simulink model "LaneFollowingController"  (R2023b)
settings: Solver=FixedStepDiscrete  StartTime=0.0  StopTime=inf  RelTol=1e-3  EnableMultiTasking=on
undefined symbols (not defined in the file): BrStatus, driver_decel, FB_decel, headwayOffset, max_ac, max_dc, PB1_decel, PB2_decel, PredictionHorizon, stopVelThreshold, time_gap, timeMargin, timeToReact, Ts
libraries: mpcadaslib x1
settings Model: Creator=The MathWorks, Inc.  LastModifiedBy=The MathWorks, Inc.
settings SolverCC: AlgebraicLoopSolver=TrustRegion  MaxZcPerStep=1
settings DataIOCC: SaveOutput=off  SaveTime=off  ReturnWorkspaceOutputs=off
settings OptimizationCC: DefaultParameterBehavior=Inlined  InlineInvariantSignals=on  EnhancedBackFolding=on  PassReuseOutputArgsAs=Individual arguments  ZeroExternalMemoryAtStartup=off  ZeroInternalMemoryAtStartup=off  EfficientFloat2IntCast=on  OptimizeBlockOrder=speed  DifferentSizesBufferReuse=on  OptimizationCustomize=off  EfficientTunableParamExpr=on
settings DebuggingCC: ParameterPrecisionLossMsg=none  ParameterTunabilityLossMsg=error  UnconnectedInputMsg=warning  UnconnectedOutputMsg=warning  UnconnectedLineMsg=warning  PregeneratedLibrarySubsystemCodeDiagnostic=none  SubsystemReferenceDiagnosticForUnitTest=warning  ArithmeticOperatorsInVariantConditions=warning
settings HardwareCC: ProdLongLongMode=on
settings ModelReferenceCC: EnableRefExpFcnMdlSchedulingChecks=on  PropagateVarSize=During execution
settings SFSimCC: SimUseLocalCustomCode=off  SimTargetLang=C++
settings RTWCC: Description=Embedded Coder  SystemTargetFile=ert.tlc  TemplateMakefile=ert_default_tmf  RTWVerbose=off  RTWUseLocalCustomCode=off  BuildConfiguration=Faster Runs  IncludeHyperlinkInReport=on  CodeExecutionProfiling=on  CodeProfilingSaveOptions=AllData  TargetLang=C++  DLArmComputeVersion=19.05
settings CodeAppCC: ForceParamTrailComments=on  IgnoreCustomStorageClasses=off  MaxIdLength=127  OperatorAnnotations=on  SimulinkDataObjDesc=on  SFDataObjDesc=on  CustomSymbolStrGlobalVar=$N$M  CustomSymbolStrType=$N$M_T  CustomSymbolStrFcn=APV_$N$M$F  CustomSymbolStrMacro=$N$M  InsertBlockDesc=on
settings ERTTargetCC: TargetLangStandard=C++03 (ISO)  GenerateSampleERTMain=on  CombineSignalStateStructs=on  CodeInterfacePackaging=C++ class  SupportVariableSizeSignals=on  CastingMode=Standards  InlinedParameterPlacement=NonHierarchical  RootIOFormat=Structure reference  ERTCustomFileTemplate=example_file_process.tlc
settings ConfigComp: CovScope=ReferencedModels  CovIncludeTopModel=off

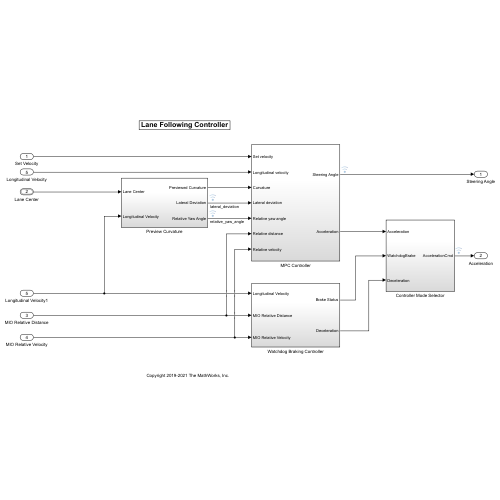
[thumbnail: Simulink's stored preview of the top-level diagram]
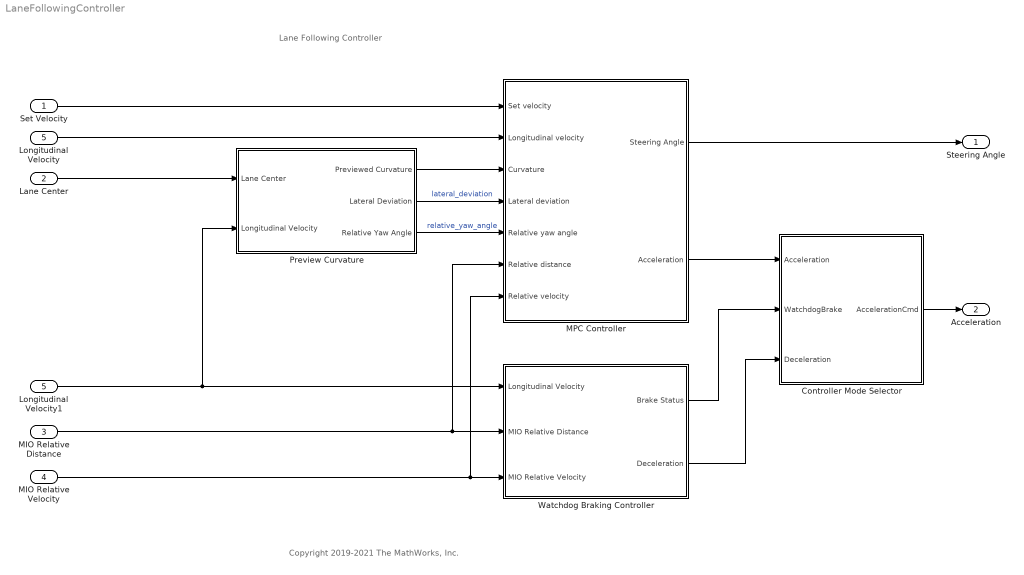
== system LaneFollowingController ==
  note: Copyright 2019-2021 The MathWorks, Inc.
  note: Lane Following Controller
  Set Velocity : Inport
  Lane Center : Inport  Port=2  OutDataTypeStr=Bus: BusLaneCenter
  MIO Relative Distance : Inport  Port=3
  MIO Relative Velocity : Inport  Port=4
  Longitudinal Velocity : Inport  Port=5
  Controller Mode Selector : Subsystem
  Longitudinal Velocity1 : InportShadow  Port=5
  MPC Controller : Subsystem
  Preview Curvature : Subsystem  VariantControl=v2
      settings: RTWFileNameOpts=Use function name
  Watchdog Braking Controller : Subsystem
  Steering Angle : Outport  PortDimensions=1  VectorParamsAs1DForOutWhenUnconnected=off
  Acceleration : Outport  Port=2  PortDimensions=1  VectorParamsAs1DForOutWhenUnconnected=off
  wires:
  Lane Center/1 -> Preview Curvature/1(Lane Center)
  Set Velocity/1 -> MPC Controller/1(Set velocity)
  Controller Mode Selector/1(AccelerationCmd) -> Acceleration/1
  Preview Curvature/3(Relative Yaw Angle) -> MPC Controller/5(Relative yaw angle)  "relative_yaw_angle"
  Longitudinal Velocity1/1 -> Preview Curvature/2(Longitudinal Velocity), Watchdog Braking Controller/1(Longitudinal Velocity)
  Watchdog Braking Controller/2(Deceleration) -> Controller Mode Selector/3(Deceleration)
  Watchdog Braking Controller/1(Brake Status) -> Controller Mode Selector/2(WatchdogBrake)
  Longitudinal Velocity/1 -> MPC Controller/2(Longitudinal velocity)
  MIO Relative Velocity/1 -> MPC Controller/7(Relative velocity), Watchdog Braking Controller/3(MIO Relative Velocity)
  Preview Curvature/2(Lateral Deviation) -> MPC Controller/4(Lateral deviation)  "lateral_deviation"
  MIO Relative Distance/1 -> Watchdog Braking Controller/2(MIO Relative Distance), MPC Controller/6(Relative distance)
  MPC Controller/1(Steering Angle) -> Steering Angle/1
  Preview Curvature/1(Previewed Curvature) -> MPC Controller/3(Curvature)
  MPC Controller/2(Acceleration) -> Controller Mode Selector/1(Acceleration)

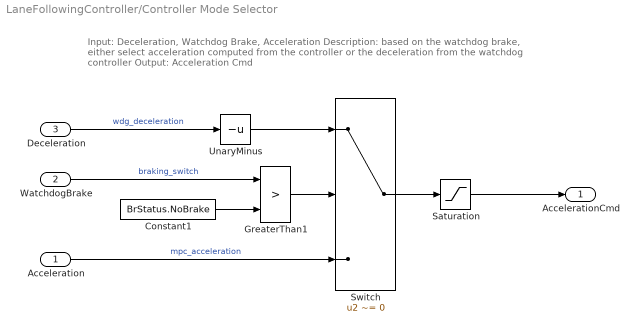
== system LaneFollowingController/Controller Mode Selector ==
  note: Input: Deceleration, Watchdog Brake, Acceleration
      | Description: based on the watchdog brake, either select acceleration computed from the controller or the deceleration from the watchdog controller
      | Output: Acceleration Cmd
  Acceleration : Inport
  WatchdogBrake : Inport  Port=2
  Deceleration : Inport  Port=3
  Constant1 : Constant  Value=BrStatus.NoBrake  OutDataTypeStr=Enum: BrStatus
  GreaterThan1 : RelationalOperator  Operator=>  RndMeth=Simplest  InputSameDT=off
  Saturation : Saturate  UpperLimit=max_ac  LowerLimit=max_dc
      settings: AttributesFormatString=|
      | %<UpperLimit>
      | %<LowerLimit>
  Switch : Switch  Criteria=u2 ~= 0  SaturateOnIntegerOverflow=off  InputSameDT=off
  UnaryMinus : UnaryMinus
  AccelerationCmd : Outport
  wires:
  Switch/1 -> Saturation/1
  WatchdogBrake/1 -> GreaterThan1/1  "braking_switch"
  UnaryMinus/1 -> Switch/1
  Deceleration/1 -> UnaryMinus/1  "wdg_deceleration"
  Saturation/1 -> AccelerationCmd/1
  Acceleration/1 -> Switch/3  "mpc_acceleration"
  Constant1/1 -> GreaterThan1/2
  GreaterThan1/1 -> Switch/2

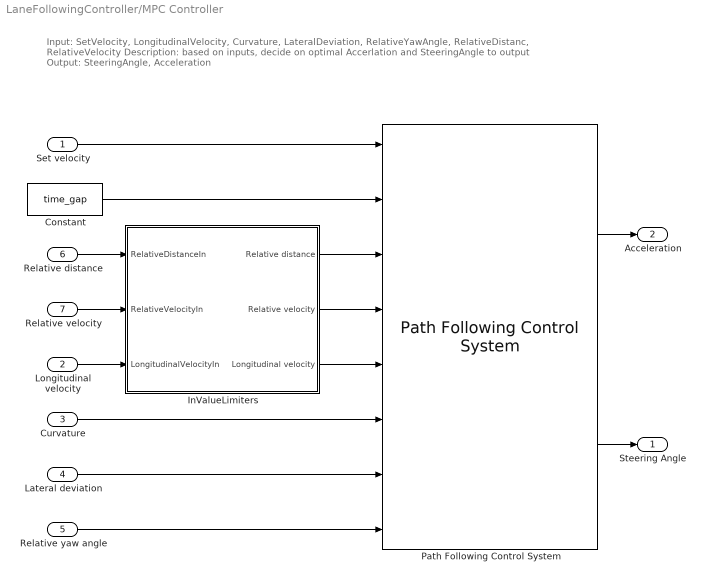
== system LaneFollowingController/MPC Controller ==
  note: Input: SetVelocity, LongitudinalVelocity, Curvature, LateralDeviation, RelativeYawAngle, RelativeDistanc, RelativeVelocity
      | Description: based on inputs, decide on optimal Accerlation and SteeringAngle to output
      | Output: SteeringAngle, Acceleration
  Set velocity : Inport
  Longitudinal velocity : Inport  Port=2
  Curvature : Inport  Port=3
  Lateral deviation : Inport  Port=4
  Relative yaw angle : Inport  Port=5
  Relative distance : Inport  Port=6
  Relative velocity : Inport  Port=7
  Constant : Constant  Value=time_gap
  InValueLimiters : Subsystem
  Path Following Control System : mpcadaslib/Path Following Control System  VariantControl=Variant2  ModelType=Use vehicle parameters  VehicleMass=m  VehicleYawInertia=Iz  LengthToFront=lf  LengthToRear=lr  FrontTireStiffness=Cf  RearTireStiffness=Cr  AccelTimeConstant=tau  EgoModelMatrixA=[-2,zeros(1,3);1,zeros(1,3);zeros(1,2),-4.4021,-12.4603;zeros(1,2),1.3913,-5.1868]  EgoModelMatrixB=[2,zeros(1,3);zeros(1,2),24.1270,15.8609]'  EgoModelMatrixC=[zeros(3,1),eye(3)]  InitialLongVel=v0_ego  TransportLag=Ts  spaceCtrl=on  DefaultSpacing=default_spacing  MinSteering=min_steer  umin_ext=off  MaxSteering=max_steer  umax_ext=off  MinAcceleration=min_ac  amin_ext=off  MaxAcceleration=max_ac  amax_ext=off  Ts=Ts  PredictionHorizon=PredictionHorizon  ControlHorizon=ControlHorizon  LongWeight=0.1  LateralWeight=1  AccelRateWeight=0.1  SteerRateWeight=0.1  suboptimal=off  maxiter=10  datatypeopt=double  optmode=off  trackmode=off
  Steering Angle : Outport  VectorParamsAs1DForOutWhenUnconnected=off
  Acceleration : Outport  Port=2  VectorParamsAs1DForOutWhenUnconnected=off
  wires:
  Constant/1 -> Path Following Control System/2
  Relative yaw angle/1 -> Path Following Control System/8
  Lateral deviation/1 -> Path Following Control System/7
  Curvature/1 -> Path Following Control System/6
  Set velocity/1 -> Path Following Control System/1
  Path Following Control System/2 -> Steering Angle/1
  Path Following Control System/1 -> Acceleration/1
  Longitudinal velocity/1 -> InValueLimiters/3(LongitudinalVelocityIn)
  Relative distance/1 -> InValueLimiters/1(RelativeDistanceIn)
  Relative velocity/1 -> InValueLimiters/2(RelativeVelocityIn)
  InValueLimiters/1(Relative distance) -> Path Following Control System/3
  InValueLimiters/2(Relative velocity) -> Path Following Control System/4
  InValueLimiters/3(Longitudinal velocity) -> Path Following Control System/5

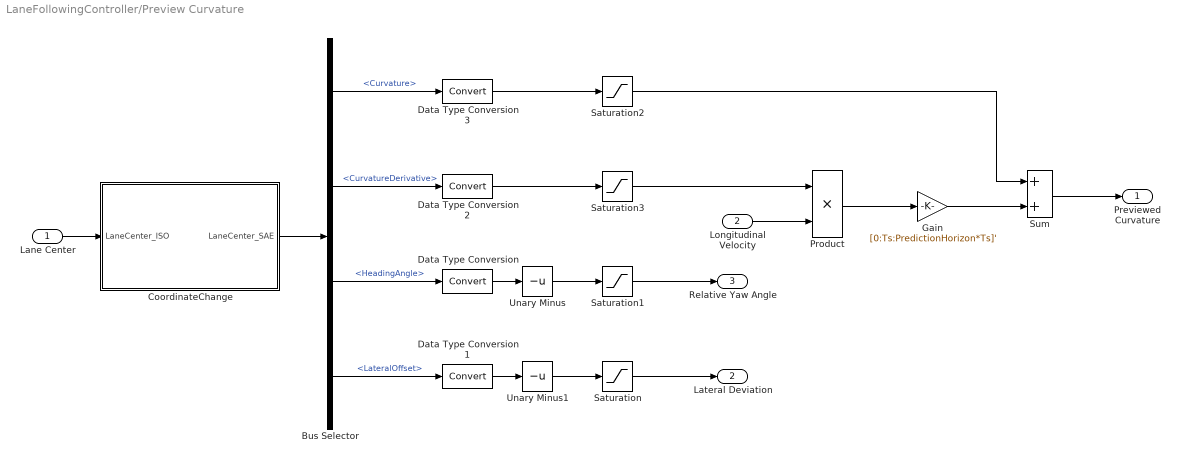
== system LaneFollowingController/Preview Curvature ==
  Lane Center : Inport
  Longitudinal Velocity : Inport  Port=2
  Bus Selector : BusSelector  OutputSignals=Curvature,CurvatureDerivative,HeadingAngle,LateralOffset
  CoordinateChange : Subsystem
  Data Type Conversion{,1..3} (4 alike) : DataTypeConversion  SaturateOnIntegerOverflow=off  RndMeth=Floor
  Gain : Gain  Gain=[0:Ts:PredictionHorizon*Ts]'
      settings: AttributesFormatString=|
      | ----------------------------------------
      | Gain = %<Gain>
  Product : Product
  Saturation : Saturate
      settings: AttributesFormatString=|
      | -------------------------------
      | UpperLimit = %<UpperLimit>
      | LowerLimit = %<LowerLimit>
  Saturation1 : Saturate  UpperLimit=0.6  LowerLimit=-0.6
      settings: AttributesFormatString=|
      | -------------------------------
      | UpperLimit = %<UpperLimit>
      | LowerLimit = %<LowerLimit>
  Saturation2 : Saturate  UpperLimit=0.15  LowerLimit=-0.15
      settings: AttributesFormatString=|
      | -------------------------------
      | UpperLimit = %<UpperLimit>
      | LowerLimit = %<LowerLimit>
  Saturation3 : Saturate  UpperLimit=0.06  LowerLimit=-0.06
      settings: AttributesFormatString=|
      | -------------------------------
      | UpperLimit = %<UpperLimit>
      | LowerLimit = %<LowerLimit>
  Sum : Sum
  Unary Minus : UnaryMinus
  Unary Minus1 : UnaryMinus
  Previewed Curvature : Outport  VectorParamsAs1DForOutWhenUnconnected=off
  Lateral Deviation : Outport  Port=2  VectorParamsAs1DForOutWhenUnconnected=off
  Relative Yaw Angle : Outport  Port=3  VectorParamsAs1DForOutWhenUnconnected=off
  wires:
  Lane Center/1 -> CoordinateChange/1(LaneCenter_ISO)
  Bus Selector/3 -> Data Type Conversion/1  "<HeadingAngle>"
  Bus Selector/4 -> Data Type Conversion1/1  "<LateralOffset>"
  Unary Minus1/1 -> Saturation/1
  Bus Selector/1 -> Data Type Conversion3/1  "<Curvature>"
  Bus Selector/2 -> Data Type Conversion2/1  "<CurvatureDerivative>"
  Longitudinal Velocity/1 -> Product/2
  Unary Minus/1 -> Saturation1/1
  Saturation/1 -> Lateral Deviation/1
  Saturation1/1 -> Relative Yaw Angle/1
  Saturation3/1 -> Product/1
  Product/1 -> Gain/1
  Sum/1 -> Previewed Curvature/1
  Gain/1 -> Sum/2
  Saturation2/1 -> Sum/1
  Data Type Conversion/1 -> Unary Minus/1
  Data Type Conversion1/1 -> Unary Minus1/1
  Data Type Conversion2/1 -> Saturation3/1
  Data Type Conversion3/1 -> Saturation2/1
  CoordinateChange/1(LaneCenter_SAE) -> Bus Selector/1

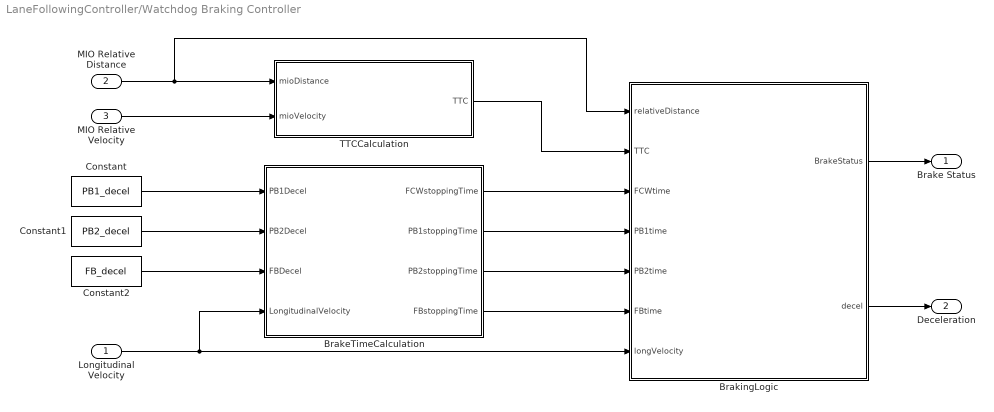
== system LaneFollowingController/Watchdog Braking Controller ==
  Longitudinal Velocity : Inport
  MIO Relative Distance : Inport  Port=2
  MIO Relative Velocity : Inport  Port=3
  BrakeTimeCalculation : Subsystem
  BrakingLogic : Subsystem
  Constant : Constant  Value=PB1_decel
  Constant1 : Constant  Value=PB2_decel
  Constant2 : Constant  Value=FB_decel
  TTCCalculation : Subsystem
  Brake Status : Outport  VectorParamsAs1DForOutWhenUnconnected=off
  Deceleration : Outport  Port=2  VectorParamsAs1DForOutWhenUnconnected=off
  wires:
  BrakingLogic/2(decel) -> Deceleration/1
  BrakingLogic/1(BrakeStatus) -> Brake Status/1
  MIO Relative Distance/1 -> BrakingLogic/1(relativeDistance), TTCCalculation/1(mioDistance)
  MIO Relative Velocity/1 -> TTCCalculation/2(mioVelocity)
  TTCCalculation/1(TTC) -> BrakingLogic/2(TTC)
  Longitudinal Velocity/1 -> BrakingLogic/7(longVelocity), BrakeTimeCalculation/4(LongitudinalVelocity)
  Constant/1 -> BrakeTimeCalculation/1(PB1Decel)
  Constant1/1 -> BrakeTimeCalculation/2(PB2Decel)
  Constant2/1 -> BrakeTimeCalculation/3(FBDecel)
  BrakeTimeCalculation/1(FCWstoppingTime) -> BrakingLogic/3(FCWtime)
  BrakeTimeCalculation/2(PB1stoppingTime) -> BrakingLogic/4(PB1time)
  BrakeTimeCalculation/3(PB2stoppingTime) -> BrakingLogic/5(PB2time)
  BrakeTimeCalculation/4(FBstoppingTime) -> BrakingLogic/6(FBtime)

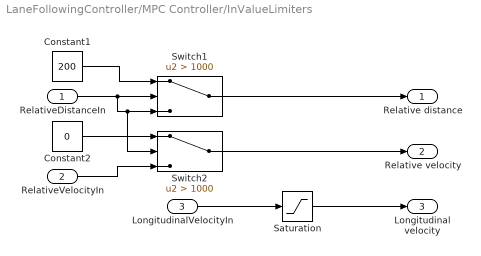
== system LaneFollowingController/MPC Controller/InValueLimiters ==
  RelativeDistanceIn : Inport
  RelativeVelocityIn : Inport  Port=2
  LongitudinalVelocityIn : Inport  Port=3
  Constant1 : Constant  Value=200
  Constant2 : Constant  Value=0
  Saturation : Saturate  UpperLimit=100  LowerLimit=0.00001
  Switch1 : Switch  Criteria=u2 > Threshold  Threshold=1000  SaturateOnIntegerOverflow=off  InputSameDT=off
  Switch2 : Switch  Criteria=u2 > Threshold  Threshold=1000  SaturateOnIntegerOverflow=off  InputSameDT=off
  Relative distance : Outport
  Relative velocity : Outport  Port=2
  Longitudinal velocity : Outport  Port=3
  wires:
  RelativeVelocityIn/1 -> Switch2/3
  Constant2/1 -> Switch2/1
  Constant1/1 -> Switch1/1
  LongitudinalVelocityIn/1 -> Saturation/1
  RelativeDistanceIn/1 -> Switch1/2, Switch1/3, Switch2/2
  Switch2/1 -> Relative velocity/1
  Switch1/1 -> Relative distance/1
  Saturation/1 -> Longitudinal velocity/1

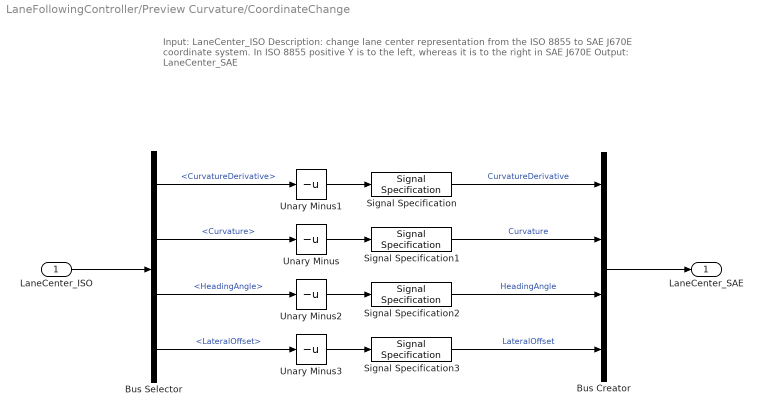
== system LaneFollowingController/Preview Curvature/CoordinateChange ==
  note: Input: LaneCenter_ISO
      | Description: change lane center representation from the ISO 8855 to SAE J670E coordinate system. In ISO 8855 positive Y is to the left, whereas it is to the right in SAE J670E
      | Output: LaneCenter_SAE
  LaneCenter_ISO : Inport
  Bus Creator : BusCreator  Inputs=4
  Bus Selector : BusSelector  OutputSignals=CurvatureDerivative,Curvature,HeadingAngle,LateralOffset
  Signal Specification : SignalSpecification  Unit=1/m^2
  Signal Specification1 : SignalSpecification  Unit=1/m
  Signal Specification2 : SignalSpecification  Unit=rad
  Signal Specification3 : SignalSpecification  Unit=m
  Unary Minus{,1..3} (4 alike) : UnaryMinus
  LaneCenter_SAE : Outport  VectorParamsAs1DForOutWhenUnconnected=off
  wires:
  Signal Specification3/1 -> Bus Creator/4  "LateralOffset"
  Signal Specification2/1 -> Bus Creator/3  "HeadingAngle"
  Signal Specification/1 -> Bus Creator/1  "CurvatureDerivative"
  Unary Minus/1 -> Signal Specification1/1
  Unary Minus3/1 -> Signal Specification3/1
  Unary Minus2/1 -> Signal Specification2/1
  Unary Minus1/1 -> Signal Specification/1
  Signal Specification1/1 -> Bus Creator/2  "Curvature"
  Bus Creator/1 -> LaneCenter_SAE/1
  Bus Selector/4 -> Unary Minus3/1  "<LateralOffset>"
  Bus Selector/3 -> Unary Minus2/1  "<HeadingAngle>"
  Bus Selector/1 -> Unary Minus1/1  "<CurvatureDerivative>"
  Bus Selector/2 -> Unary Minus/1  "<Curvature>"
  LaneCenter_ISO/1 -> Bus Selector/1

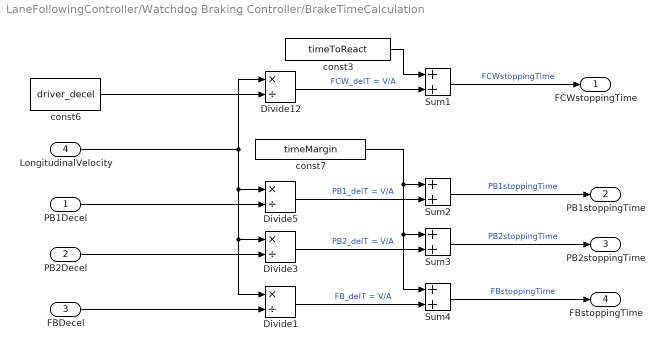
== system LaneFollowingController/Watchdog Braking Controller/BrakeTimeCalculation ==
  PB1Decel : Inport
  PB2Decel : Inport  Port=2
  FBDecel : Inport  Port=3
  LongitudinalVelocity : Inport  Port=4
  Divide{1,3,5,12} (4 alike) : Product  Inputs=*/
  Sum{1..4} (4 alike) : Sum
  const3 : Constant  Value=timeToReact  SampleTime=-1
  const6 : Constant  Value=driver_decel  SampleTime=-1
  const7 : Constant  Value=timeMargin  SampleTime=-1
  FCWstoppingTime : Outport
  PB1stoppingTime : Outport  Port=2
  PB2stoppingTime : Outport  Port=3
  FBstoppingTime : Outport  Port=4
  wires:
  Sum2/1 -> PB1stoppingTime/1  "PB1stoppingTime"
  const7/1 -> Sum3/1, Sum4/1, Sum2/1
  Divide12/1 -> Sum1/2  "FCW_delT = V/A"
  LongitudinalVelocity/1 -> Divide3/1, Divide1/1, Divide5/1, Divide12/1
  PB2Decel/1 -> Divide3/2
  Divide1/1 -> Sum4/2  "FB_delT = V/A"
  Divide3/1 -> Sum3/2  "PB2_delT = V/A"
  Divide5/1 -> Sum2/2  "PB1_delT = V/A"
  const3/1 -> Sum1/1
  FBDecel/1 -> Divide1/2
  const6/1 -> Divide12/2
  PB1Decel/1 -> Divide5/2
  Sum4/1 -> FBstoppingTime/1  "FBstoppingTime"
  Sum3/1 -> PB2stoppingTime/1  "PB2stoppingTime"
  Sum1/1 -> FCWstoppingTime/1  "FCWstoppingTime"

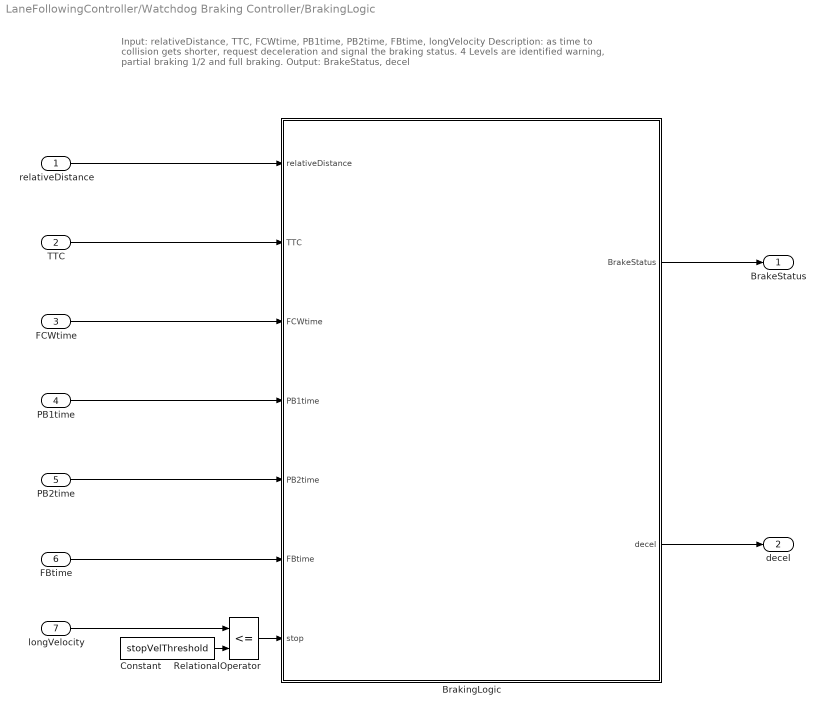
== system LaneFollowingController/Watchdog Braking Controller/BrakingLogic ==
  note: Input: relativeDistance, TTC, FCWtime, PB1time, PB2time, FBtime, longVelocity
      | Description: as time to collision gets shorter, request deceleration and signal the braking status. 4 Levels are identified warning, partial braking 1/2 and full braking.
      | Output: BrakeStatus, decel
  relativeDistance : Inport
  TTC : Inport  Port=2
  FCWtime : Inport  Port=3
  PB1time : Inport  Port=4
  PB2time : Inport  Port=5
  FBtime : Inport  Port=6
  longVelocity : Inport  Port=7
  BrakingLogic : Stateflow chart  TreatAsAtomicUnit=on
  Constant : Constant  Value=stopVelThreshold  SampleTime=Ts
      settings: AttributesFormatString=%<SampleTime>
  RelationalOperator : RelationalOperator  Operator=<=  RndMeth=Simplest  InputSameDT=off
  BrakeStatus : Outport
  decel : Outport  Port=2
  wires:
  RelationalOperator/1 -> BrakingLogic/7(stop)
  relativeDistance/1 -> BrakingLogic/1(relativeDistance)
  BrakingLogic/2(decel) -> decel/1
  TTC/1 -> BrakingLogic/2(TTC)
  PB1time/1 -> BrakingLogic/4(PB1time)
  longVelocity/1 -> RelationalOperator/1
  FBtime/1 -> BrakingLogic/6(FBtime)
  FCWtime/1 -> BrakingLogic/3(FCWtime)
  BrakingLogic/1(BrakeStatus) -> BrakeStatus/1
  PB2time/1 -> BrakingLogic/5(PB2time)
  Constant/1 -> RelationalOperator/2

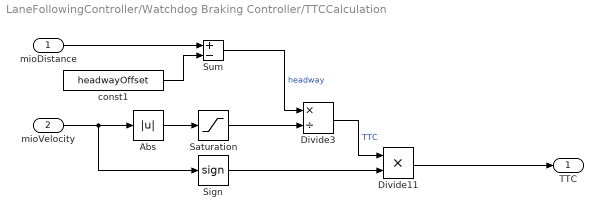
== system LaneFollowingController/Watchdog Braking Controller/TTCCalculation ==
  mioDistance : Inport
  mioVelocity : Inport  Port=2
  Abs : Abs  SaturateOnIntegerOverflow=off
  Divide11 : Product  Inputs=**
  Divide3 : Product  Inputs=*/
  Saturation : Saturate  UpperLimit=100  LowerLimit=0.01
  Sign : Signum
  Sum : Sum  Inputs=+-
  const1 : Constant  Value=headwayOffset  SampleTime=-1
  TTC : Outport  VectorParamsAs1DForOutWhenUnconnected=off
  wires:
  mioVelocity/1 -> Sign/1, Abs/1
  mioDistance/1 -> Sum/1
  Divide3/1 -> Divide11/1  "TTC"
  const1/1 -> Sum/2
  Sum/1 -> Divide3/1  "headway"
  Abs/1 -> Saturation/1
  Saturation/1 -> Divide3/2
  Sign/1 -> Divide11/2
  Divide11/1 -> TTC/1

== stateflow chart LaneFollowingController/Watchdog Braking Controller/BrakingLogic/BrakingLogic ==
  state Default
    entry:
    BrakeStatus = BrStatus.NoBrake;
    decel = Default_decel;
  state FCW
    entry:
    BrakeStatus = BrStatus.NoBrake;
    decel = Default_decel;
  state Partial_Braking1
    entry:
    BrakeStatus = BrStatus.PB1Brake;
    decel = PB1_decel;
  state Partial_Braking2
    entry:
    BrakeStatus =BrStatus.PB2Brake;
    decel = PB2_decel;
  state Full_Braking
    entry:
    BrakeStatus = BrStatus.FBrake;
    decel = FB_decel;
  (default) -> Default
  Default -> (junction 114) [order 2]
  (junction 114) -> Full_Braking : [relativeDistance < default_spacing]
  (junction 95) -> Default
  Full_Braking -> (junction 95) : [stop && TTC>double(0) && relativeDistance > default_spacing ]
  (junction 101) -> Default
  (junction 103) -> (junction 101) : [stop]
  (junction 97) -> Default
  (junction 99) -> (junction 97) : [stop]
  Default -> FCW [order 1] : [(abs(TTC)<FCWtime) && TTC<double(0)]
  FCW -> Default [order 2] : [abs(TTC)>=TimeFactor*FCWtime]
  FCW -> Partial_Braking1 [order 1] : [(abs(TTC) < PB1time) && TTC<double(0)]
  Partial_Braking1 -> (junction 99) [order 2]
  Partial_Braking1 -> Partial_Braking2 [order 1] : [(abs(TTC) < PB2time) && TTC<double(0)]
  Partial_Braking2 -> (junction 103) [order 2]
  Partial_Braking2 -> Full_Braking [order 1] : [(abs(TTC) < FBtime) && TTC<double(0)]
  data: relativeDistance input; TTC input; FCWtime input; PB1time input; PB2time input; FBtime input; BrakeStatus output; decel output; stop input boolean; FB_decel constant double =FB_decel; PB2_decel constant double =PB2_decel; Default_decel constant double =Default_decel; TimeFactor constant double =TimeFactor; PB1_decel constant double =PB1_decel; default_spacing constant double =default_spacing
